simulink model "CACC_Model_5V"  (R2019b)
settings: Solver=ode45  StartTime=0.0  StopTime=20  FixedStep=0.01  MaxStep=0.001  RelTol=1e-3  EnableMultiTasking=on
InitFcn:
  | %% CACC Simulation Parameters
  | %% by M.Tolga EMIRLER ITU MEKAR
undefined symbols (not defined in the file): sigbuilder_block
libraries: simulink_need_slupdate x5, simulink x1
settings Model: Creator=Tolga  LastModifiedBy=subhajyotisarkar
settings DataIOCC: LimitDataPoints=on  SaveFormat=Array  SignalLoggingSaveFormat=ModelDataLogs  ReturnWorkspaceOutputs=off
settings OptimizationCC: ExpressionDepthLimit=2147483647  LifeSpan=inf
settings DebuggingCC: UnderspecifiedInitializationDetection=Classic  MergeDetectMultiDrivingBlocksExec=none  SolverPrmCheckMsg=warning  FcnCallInpInsideContextMsg=warning  StateNameClashWarn=warning  SFUnexpectedBacktrackingDiag=warning  SFNoUnconditionalDefaultTransitionDiag=warning  SFExecutionAtInitializationDiag=none  ArithmeticOperatorsInVariantConditions=warning
settings HardwareCC: ProdBitPerPointer=32  ProdBitPerSizeT=32  ProdBitPerPtrDiffT=32  ProdLargestAtomicFloat=None  ProdIntDivRoundTo=Undefined  ProdEndianess=Unspecified  ProdWordSize=32  ProdHWDeviceType=32-bit Generic
settings ModelReferenceCC: PropagateSignalLabelsOutOfModel=off
settings SFSimCC: SimUseLocalCustomCode=off  CustomCodeUndefinedFunction=UseInterfaceOnly
settings RTWCC: RTWUseLocalCustomCode=off
settings CodeAppCC: StateflowObjectComments=on
settings GRTTargetCC: TargetLangStandard=C89/C90 (ANSI)  GeneratePreprocessorConditionals=Disable all  CombineOutputUpdateFcns=off  GRTInterface=on
settings ConfigComp: CovMetricSettings=dw  CovHtmlReporting=on  CovSaveCumulativeToWorkspaceVar=on  CovSaveSingleToWorkspaceVar=on  CovExternalEMLEnable=off  CovSFcnEnable=off

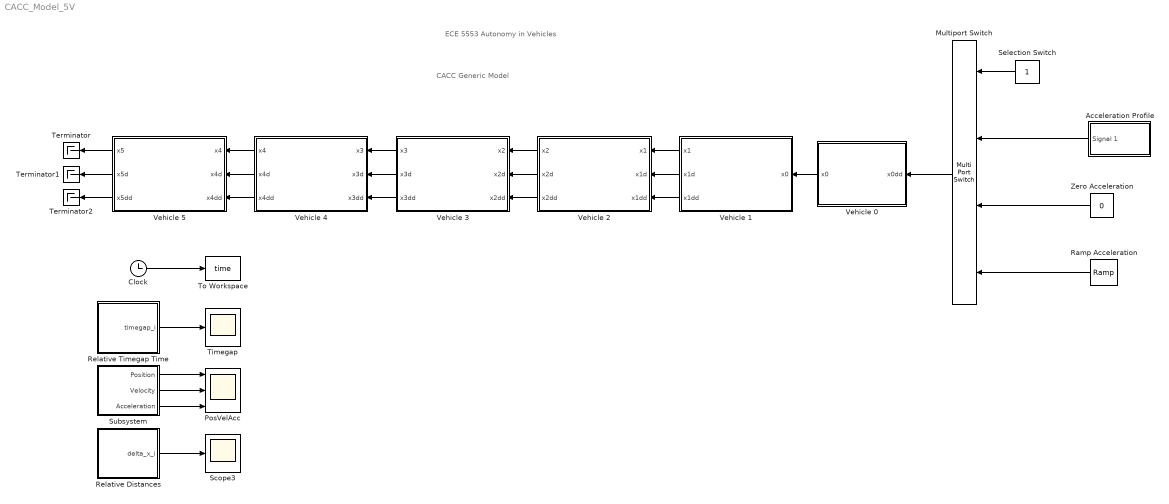
== system CACC_Model_5V ==
  note: ECE 5553 Autonomy in Vehicles
  note: CACC Generic Model
  Acceleration Profile : Subsystem  Tag=STV Subsys  LoadFcn=sigbuilder_block('load');  StartFcn=sigbuilder_block('start');  StopFcn=sigbuilder_block('stop');  ClipboardFcn=sigbuilder_block('clipboard');  mask(Sigbuilder block){tuvar=[0:10]}
      mask help: Sigbuilder GUI
      mask init:
      | if ~strcmp(get_param(bdroot(gcbh),'SimulationStatus'),'stopped') tuvar = sigbuilder_block('maskInit'); end
      settings: CopyFcn=sigbuilder_block('copy');  DeleteFcn=sigbuilder_block('delete');  ModelCloseFcn=sigbuilder_block('modelClose');  PreSaveFcn=sigbuilder_block('preSave');  PauseFcn=sigbuilder_block('pause')  ContinueFcn=sigbuilder_block('continue')  NameChangeFcn=sigbuilder_block('namechange');  OpenFcn=sigbuilder_block('open',[386.25 100.5 510.75 487.5 ]);  CloseFcn=sigbuilder_block('close');
      mask Display: plot(0, 0, 100, 100,[2, 2, 32, 32, 2], [68, 8, 8, 68, 68],[32, 2], [38, 38], [32, 19, 2],[53, 60, 44], [32, 17, 17, 2],[16, 16, 31, 31]);txt = getActiveGroup(gcbh);text(2, 100, txt,'verticalAlignment', 'top');
  Clock : Clock
  Multiport Switch : MultiPortSwitch
  PosVelAcc : Scope  NumInputPorts=3
  Ramp Acceleration : simulink/Sources/Ramp  slope=1  start=0  InitialOutput=40
  Relative Distances : Subsystem
  Relative Timegap Time : Subsystem
  Scope3 : Scope
  Selection Switch : Constant
  Subsystem : Subsystem
  Terminator : Terminator
  Terminator1 : Terminator
  Terminator2 : Terminator
  Timegap : Scope
  To Workspace : ToWorkspace  VariableName=time  SampleTime=-1
  Vehicle 0 : Subsystem  mask(INPUT BLOCK){x0in=250, V0in=25}
      mask prompts: x0in "Initial position (x0in)"; V0in "Initial velocity (V0in)"
      mask help: This block defines the input. Input (or disturbance) is the acceleration.
      mask Display:
      | disp('Input')
      | port_label('input',1,'a0')
      | port_label('output',1,'x0')
  Vehicle 1 : Subsystem  mask(VEHICLE #1 (GCDC Vehicle)){kG1=1.0, T1=0.5, phi1=0.1, theta1=0.3, hd1=0.6, L1=5, r1=30, x1in=200, V1in=25, CACC1=1, wK1=2.4}
      mask prompts: kG1 "Vehicle Model Gain (kG1)"; T1 "Vehicle Time Constant (T1)"; phi1 "Actuator (Internal) Delay (phi1) [s]"; theta1 "Communication System Delay (theta1) [s]"; hd1 "Headway time (hd1) [s]"; L1 "Vehicle length (L1) [m]"; r1 "Distance at standstill (r1) [m]"; x1in "Initial vehicle position (x1in) [m]"; V1in "Initial vehicle velocity (V1in) [m/sec]"; CACC1 "CACC On/Off [0 or 1]"; wK1 "Controller Gain (wK1)"
      mask help: Parameters for vehicle 1
      mask Display:
      | disp('Vehicle 1')
      | port_label('input',1,'x0')
      | port_label('output',1,'x1')
      | port_label('output',2,'V1')
      | port_label('output',3,'a1')
  Vehicle 2 : Subsystem  mask(VEHICLE #2){kG2=1.0, T2=0.5, phi2=0.1, theta2=0.3, hd2=0.6, L2=5, r2=30, x2in=150, V2in=25, CACC2=0, wK2=2.4}
      mask prompts: kG2 "Vehicle Model Gain (kG2)"; T2 "Vehicle Time Constant (T2)"; phi2 "Actuator (Internal) Delay (phi2) [s]"; theta2 "Communication System Delay (theta2) [s]"; hd2 "Headway time (hd2) [s]"; L2 "Vehicle length (L2) [m]"; r2 "Distance at standstill (r2) [m]"; x2in "Initial vehicle position (x2in) [m]"; V2in "Initial vehicle velocity (V2in) [m/sec]"; CACC2 "CACC On/Off [0 or 1]"; wK2 "Controller Gain (wK2)"
      mask help: Parameters for vehicle 2
      mask Display:
      | disp('Vehicle 2')
      | port_label('input',1,'x1')
      | port_label('input',2,'V1')
      | port_label('input',3,'a1')
      | port_label('output',1,'x2')
      | port_label('output',2,'V2')
      | port_label('output',3,'a2')
  Vehicle 3 : Subsystem  mask(VEHICLE #3){kG3=1.0, T3=0.5, phi3=0.1, theta3=0.3, hd3=0.6, L3=5, r3=30, x3in=100, V3in=25, CACC3=0, wK3=2.4}
      mask prompts: kG3 "Vehicle Model Gain (kG3)"; T3 "Vehicle Time Constant (T3)"; phi3 "Actuator (Internal) Delay (phi3) [s]"; theta3 "Communication System Delay (theta3) [s]"; hd3 "Headway time (hd3) [s]"; L3 "Vehicle length (L3) [m]"; r3 "Distance at standstill (r3) [m]"; x3in "Initial vehicle position (x3in) [m]"; V3in "Initial vehicle velocity (V3in) [m/sec]"; CACC3 "CACC On/Off [0 or 1]"; wK3 "Controller Gain (wK3)"
      mask help: Parameters for vehicle 3
      mask Display:
      | disp('Vehicle 3')
      | port_label('input',1,'x2')
      | port_label('input',2,'V2')
      | port_label('input',3,'a2')
      | port_label('output',1,'x3')
      | port_label('output',2,'V3')
      | port_label('output',3,'a3')
  Vehicle 4 : Subsystem  mask(VEHICLE #4){kG4=1.0, T4=0.5, phi4=0.1, theta4=0.3, hd4=0.6, L4=5, r4=30, x4in=50, V4in=25, CACC4=0, wK4=2.4}
      mask prompts: kG4 "Vehicle Model Gain (kG4)"; T4 "Vehicle Time Constant (T4)"; phi4 "Actuator (Internal) Delay (phi4) [s]"; theta4 "Communication System Delay (theta4) [s]"; hd4 "Headway time (hd4) [s]"; L4 "Vehicle length (L4) [m]"; r4 "Distance at standstill (r4) [m]"; x4in "Initial vehicle position (x4in) [m]"; V4in "Initial vehicle velocity (V4in) [m/sec]"; CACC4 "CACC On/Off [0 or 1]"; wK4 "Controller Gain (wK4)"
      mask help: Parameters for vehicle 4
      mask Display:
      | disp('Vehicle 4')
      | port_label('input',1,'x3')
      | port_label('input',2,'V3')
      | port_label('input',3,'a3')
      | port_label('output',1,'x4')
      | port_label('output',2,'V4')
      | port_label('output',3,'a4')
  Vehicle 5 : Subsystem  mask(VEHICLE #5){kG5=1.0, T5=0.5, phi5=0.1, theta5=0.3, hd5=0.6, L5=5, r5=30, x5in=0, V5in=25, CACC5=0, wK5=2.4}
      mask prompts: kG5 "Vehicle Model Gain (kG5)"; T5 "Vehicle Time Constant (T5)"; phi5 "Actuator (Internal) Delay (phi5) [s]"; theta5 "Communication System Delay (theta5) [s]"; hd5 "Headway time (hd5) [s]"; L5 "Vehicle length (L5) [m]"; r5 "Distance at standstill (r5) [m]"; x5in "Initial vehicle position (x5in) [m]"; V5in "Initial vehicle velocity (V5in) [m/sec]"; CACC5 "CACC On/Off [0 or 1]"; wK5 "Controller Gain (wK5)"
      mask help: Parameters for vehicle 5
      mask Display:
      | disp('Vehicle 5')
      | port_label('input',1,'x4')
      | port_label('input',2,'V4')
      | port_label('input',3,'a4')
      | port_label('output',1,'x5')
      | port_label('output',2,'V5')
      | port_label('output',3,'a5')
  Zero Acceleration : Constant  Value=0
  wires:
  Clock/1 -> To Workspace/1
  Relative Distances/1(delta_x_i) -> Scope3/1
  Vehicle 2/1(x2) -> Vehicle 3/1(x2)
  Vehicle 2/2(x2d) -> Vehicle 3/2(x2d)
  Vehicle 4/1(x4) -> Vehicle 5/1(x4)
  Vehicle 4/2(x4d) -> Vehicle 5/2(x4d)
  Vehicle 4/3(x4dd) -> Vehicle 5/3(x4dd)
  Vehicle 3/1(x3) -> Vehicle 4/1(x3)
  Vehicle 3/2(x3d) -> Vehicle 4/2(x3d)
  Vehicle 1/1(x1) -> Vehicle 2/1(x1)
  Vehicle 1/2(x1d) -> Vehicle 2/2(x1d)
  Vehicle 0/1(x0) -> Vehicle 1/1(x0)
  Ramp Acceleration/1 -> Multiport Switch/4
  Vehicle 1/3(x1dd) -> Vehicle 2/3(x1dd)
  Vehicle 2/3(x2dd) -> Vehicle 3/3(x2dd)
  Vehicle 3/3(x3dd) -> Vehicle 4/3(x3dd)
  Acceleration Profile/1(Signal 1) -> Multiport Switch/2
  Zero Acceleration/1 -> Multiport Switch/3
  Vehicle 5/1(x5) -> Terminator/1
  Vehicle 5/2(x5d) -> Terminator1/1
  Vehicle 5/3(x5dd) -> Terminator2/1
  Relative Timegap Time/1(timegap_i) -> Timegap/1
  Selection Switch/1 -> Multiport Switch/1
  Multiport Switch/1 -> Vehicle 0/1(x0dd)
  Subsystem/1(Position) -> PosVelAcc/1
  Subsystem/2(Velocity) -> PosVelAcc/2
  Subsystem/3(Acceleration) -> PosVelAcc/3

== system CACC_Model_5V/Acceleration Profile ==
  Demux : Demux  Tag=STV Demux  Outputs=1
  FromWs : FromWorkspace  Tag=STV FromWs  VariableName=tuvar  SampleTime=0
      SigBuilderData=|
      | common.afterFinalStr = 'Extrapolate'
      | common.sampleTime = 0
      | dataSet.timeRange = [0 50]
      | dataSet.name = 'Group 1'
      | sbobj.Groups.Name = 'Group 1'
      | sbobj.Groups.Signals.Name = 'Signal 1'
      | sbobj.Groups.Signals.XData = [0 5 10 15 25 30 35 40 50]
      | sbobj.Groups.Signals.YData = [0 1 1 0 0 -1 -1 0 0]
      | sbobj.Groups.TimeRange = [0 50]
  Signal 1 : Outport  Tag=STV Outport  VectorParamsAs1DForOutWhenUnconnected=off
  wires:
  Demux/1 -> Signal 1/1
  FromWs/1 -> Demux/1

== system CACC_Model_5V/Relative Distances ==
  Mux2 : Mux
  Sum{,1..3} (4 alike) : Sum  Inputs=|+-
  delta_x_i : Outport  VectorParamsAs1DForOutWhenUnconnected=off
  wires:
  [x1] -> Sum/1
  [x2] -> Sum/2, Sum1/1
  [x3] -> Sum1/2, Sum2/1
  Sum/1 -> Mux2/1
  Sum1/1 -> Mux2/2
  Sum2/1 -> Mux2/3
  Mux2/1 -> delta_x_i/1
  Sum3/1 -> Mux2/4
  [x5] -> Sum3/2
  [x4] -> Sum3/1, Sum2/2

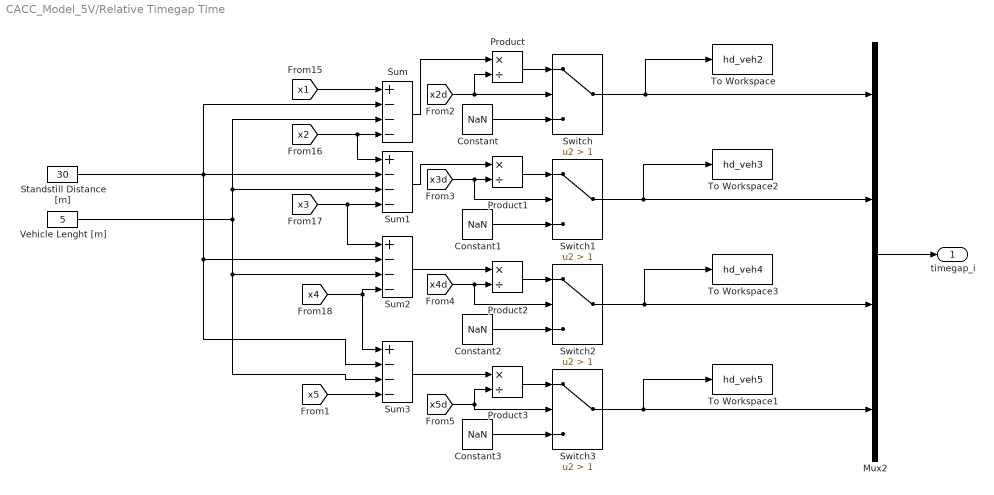
== system CACC_Model_5V/Relative Timegap Time ==
  Constant{,1..3} (4 alike) : Constant  Value=NaN
  Mux2 : Mux
  Product{,1..3} (4 alike) : Product  Inputs=*/
  Standstill Distance [m] : Constant  Value=30
  Sum{,1..3} (4 alike) : Sum  Inputs=+---
  Switch{,1..3} (4 alike) : Switch  Criteria=u2 > Threshold  Threshold=1
  To Workspace : ToWorkspace  VariableName=hd_veh2  SampleTime=-1
  To Workspace1 : ToWorkspace  VariableName=hd_veh5  SampleTime=-1
  To Workspace2 : ToWorkspace  VariableName=hd_veh3  SampleTime=-1
  To Workspace3 : ToWorkspace  VariableName=hd_veh4  SampleTime=-1
  Vehicle Lenght [m] : Constant  Value=5
  timegap_i : Outport  VectorParamsAs1DForOutWhenUnconnected=off
  wires:
  [x4] -> Sum3/1, Sum2/4
  [x5] -> Sum3/4
  Mux2/1 -> timegap_i/1
  Sum/1 -> Product/1
  [x3] -> Sum2/1, Sum1/4
  [x2] -> Sum1/1, Sum/4
  [x1] -> Sum/1
  Product/1 -> Switch/1
  [x2d] -> Switch/2, Product/2
  Constant/1 -> Switch/3
  Switch/1 -> Mux2/1, To Workspace/1
  Constant1/1 -> Switch1/3
  [x3d] -> Switch1/2, Product1/2
  Product1/1 -> Switch1/1
  Sum1/1 -> Product1/1
  Sum2/1 -> Product2/1
  Product2/1 -> Switch2/1
  [x4d] -> Switch2/2, Product2/2
  Constant2/1 -> Switch2/3
  Constant3/1 -> Switch3/3
  [x5d] -> Switch3/2, Product3/2
  Product3/1 -> Switch3/1
  Sum3/1 -> Product3/1
  Switch1/1 -> To Workspace2/1, Mux2/2
  Switch3/1 -> To Workspace1/1, Mux2/4
  Switch2/1 -> To Workspace3/1, Mux2/3
  Standstill Distance [m]/1 -> Sum3/2, Sum2/2, Sum1/2, Sum/2
  Vehicle Lenght [m]/1 -> Sum3/3, Sum2/3, Sum1/3, Sum/3

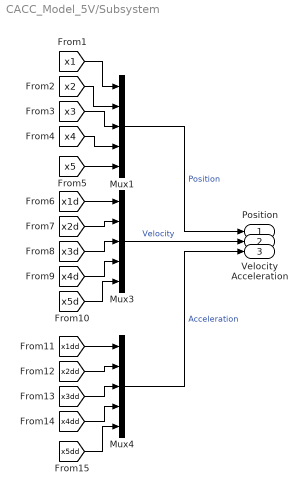
== system CACC_Model_5V/Subsystem ==
  Mux1 : Mux  Inputs=5
  Mux3 : Mux  Inputs=5
  Mux4 : Mux  Inputs=5
  Position : Outport  VectorParamsAs1DForOutWhenUnconnected=off
  Velocity : Outport  Port=2  VectorParamsAs1DForOutWhenUnconnected=off
  Acceleration : Outport  Port=3  VectorParamsAs1DForOutWhenUnconnected=off
  wires:
  Mux1/1 -> Position/1  "Position"
  Mux3/1 -> Velocity/1  "Velocity"
  Mux4/1 -> Acceleration/1  "Acceleration"
  [x2dd] -> Mux4/2
  [x2] -> Mux1/2
  [x1dd] -> Mux4/1
  [x4d] -> Mux3/4
  [x1] -> Mux1/1
  [x4] -> Mux1/4
  [x1d] -> Mux3/1
  [x3d] -> Mux3/3
  [x4dd] -> Mux4/4
  [x3] -> Mux1/3
  [x2d] -> Mux3/2
  [x3dd] -> Mux4/3
  [x5dd] -> Mux4/5
  [x5d] -> Mux3/5
  [x5] -> Mux1/5

== system CACC_Model_5V/Vehicle 0 ==
  x0dd : Inport
  Integrator : Integrator  InitialCondition=V0in
  Integrator1 : Integrator  InitialCondition=x0in
  To Workspace : ToWorkspace  VariableName=x0dd  SampleTime=-1
  To Workspace1 : ToWorkspace  VariableName=x0d  SampleTime=-1
  To Workspace2 : ToWorkspace  VariableName=x0  SampleTime=-1
  x0 : Outport  VectorParamsAs1DForOutWhenUnconnected=off
  wires:
  Integrator/1 -> Integrator1/1, To Workspace1/1
  x0dd/1 -> Integrator/1, To Workspace/1
  Integrator1/1 -> x0/1, To Workspace2/1

== system CACC_Model_5V/Vehicle 1 ==
  note: a
  note: e1
  note: Spacing Error
  x0 : Inport
  ACC Signal Measurement Delay : TransportDelay  DelayTime=0
  PD Controller : simulink_need_slupdate/PID Controller  P=wK1^2  I=0  D=wK1
      settings: SourceProductName=Simulink
  Spacing Policy : Subsystem
  Vehicle 1 : Subsystem
  x1 : Outport  VectorParamsAs1DForOutWhenUnconnected=off
  x1d : Outport  Port=2  VectorParamsAs1DForOutWhenUnconnected=off
  x1dd : Outport  Port=3  VectorParamsAs1DForOutWhenUnconnected=off
  wires:
  Vehicle 1/3(x1dd) -> x1dd/1
  Vehicle 1/2(x1d) -> x1d/1, Spacing Policy/3(x2d)
  Vehicle 1/1(x1) -> x1/1, Spacing Policy/2(x1)
  Spacing Policy/1(e1) -> PD Controller/1
  x0/1 -> ACC Signal Measurement Delay/1
  PD Controller/1 -> Vehicle 1/1(a_cont1)
  ACC Signal Measurement Delay/1 -> Spacing Policy/1(x0)

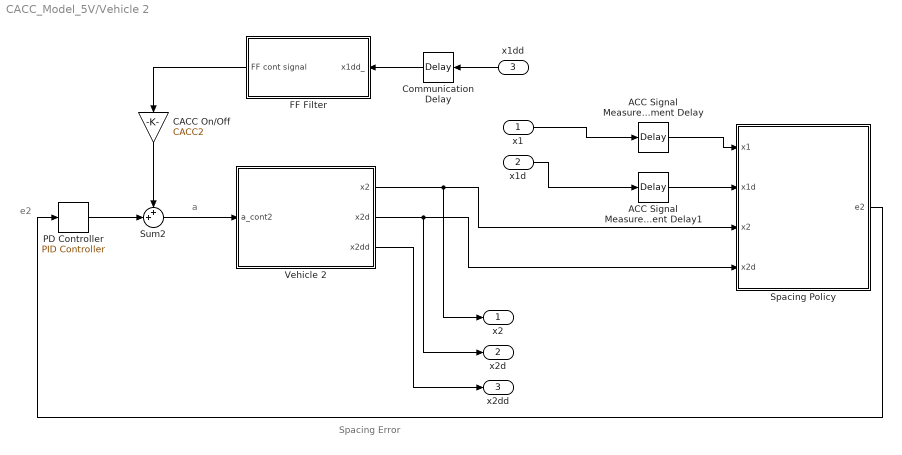
== system CACC_Model_5V/Vehicle 2 ==
  note: Spacing Error
  note: e2
  note: a
  x1 : Inport
  x1d : Inport  Port=2
  x1dd : Inport  Port=3
  ACC Signal Measurement Delay : TransportDelay  DelayTime=0
  ACC Signal Measurement Delay1 : TransportDelay  DelayTime=0
  CACC On/Off : Gain  Gain=CACC2
  Communication Delay : TransportDelay  DelayTime=theta2
  FF Filter : Subsystem
  PD Controller : simulink_need_slupdate/PID Controller  P=wK2*wK2  I=0  D=wK2
      settings: SourceProductName=Simulink
  Spacing Policy : Subsystem
  Sum2 : Sum  Inputs=++|
  Vehicle 2 : Subsystem
  x2 : Outport  VectorParamsAs1DForOutWhenUnconnected=off
  x2d : Outport  Port=2  VectorParamsAs1DForOutWhenUnconnected=off
  x2dd : Outport  Port=3  VectorParamsAs1DForOutWhenUnconnected=off
  wires:
  PD Controller/1 -> Sum2/2
  Sum2/1 -> Vehicle 2/1(a_cont2)
  x1dd/1 -> Communication Delay/1
  Communication Delay/1 -> FF Filter/1(x1dd_)
  x1/1 -> ACC Signal Measurement Delay/1
  Spacing Policy/1(e2) -> PD Controller/1
  x1d/1 -> ACC Signal Measurement Delay1/1
  Vehicle 2/1(x2) -> Spacing Policy/3(x2), x2/1
  Vehicle 2/2(x2d) -> Spacing Policy/4(x2d), x2d/1
  Vehicle 2/3(x2dd) -> x2dd/1
  FF Filter/1(FF cont signal) -> CACC On/Off/1
  CACC On/Off/1 -> Sum2/1
  ACC Signal Measurement Delay/1 -> Spacing Policy/1(x1)
  ACC Signal Measurement Delay1/1 -> Spacing Policy/2(x1d)

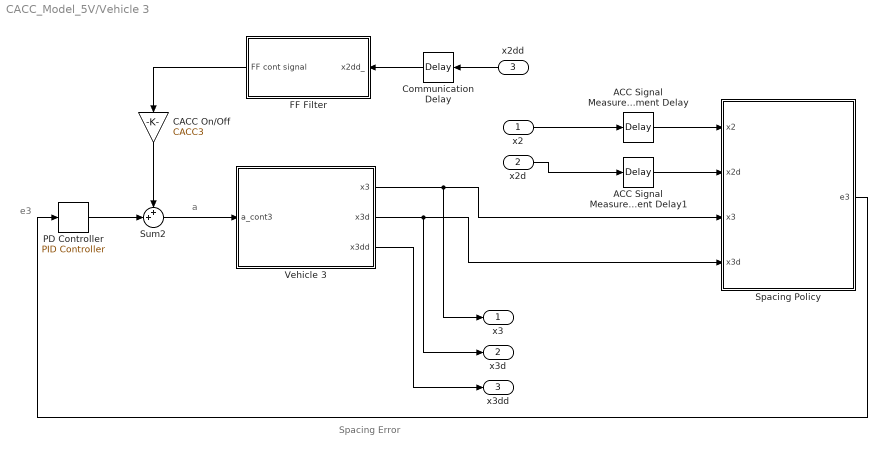
== system CACC_Model_5V/Vehicle 3 ==
  note: a
  note: e3
  note: Spacing Error
  x2 : Inport
  x2d : Inport  Port=2
  x2dd : Inport  Port=3
  ACC Signal Measurement Delay : TransportDelay  DelayTime=0
  ACC Signal Measurement Delay1 : TransportDelay  DelayTime=0
  CACC On/Off : Gain  Gain=CACC3
  Communication Delay : TransportDelay  DelayTime=theta3
  FF Filter : Subsystem
  PD Controller : simulink_need_slupdate/PID Controller  P=wK3*wK3  I=0  D=wK3
      settings: SourceProductName=Simulink
  Spacing Policy : Subsystem
  Sum2 : Sum  Inputs=++|
  Vehicle 3 : Subsystem
  x3 : Outport  VectorParamsAs1DForOutWhenUnconnected=off
  x3d : Outport  Port=2  VectorParamsAs1DForOutWhenUnconnected=off
  x3dd : Outport  Port=3  VectorParamsAs1DForOutWhenUnconnected=off
  wires:
  CACC On/Off/1 -> Sum2/1
  FF Filter/1(FF cont signal) -> CACC On/Off/1
  Vehicle 3/3(x3dd) -> x3dd/1
  Vehicle 3/2(x3d) -> x3d/1, Spacing Policy/4(x3d)
  Vehicle 3/1(x3) -> x3/1, Spacing Policy/3(x3)
  x2d/1 -> ACC Signal Measurement Delay1/1
  Spacing Policy/1(e3) -> PD Controller/1
  x2/1 -> ACC Signal Measurement Delay/1
  Communication Delay/1 -> FF Filter/1(x2dd_)
  x2dd/1 -> Communication Delay/1
  Sum2/1 -> Vehicle 3/1(a_cont3)
  PD Controller/1 -> Sum2/2
  ACC Signal Measurement Delay/1 -> Spacing Policy/1(x2)
  ACC Signal Measurement Delay1/1 -> Spacing Policy/2(x2d)

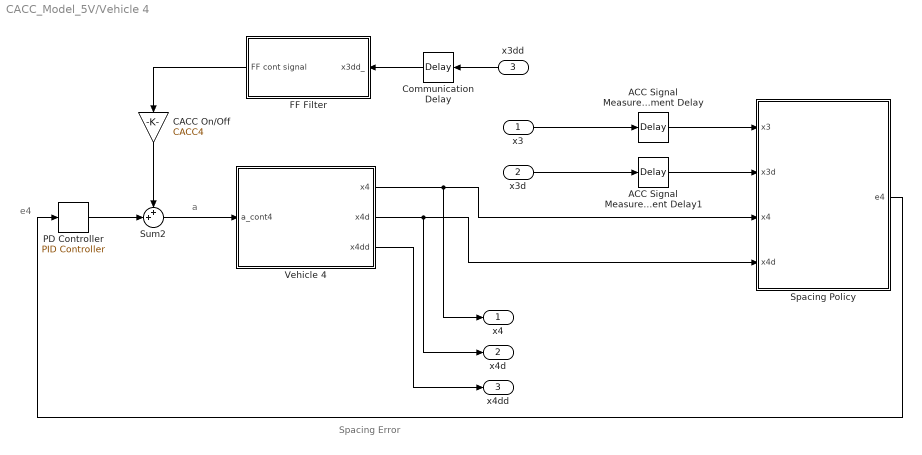
== system CACC_Model_5V/Vehicle 4 ==
  note: a
  note: e4
  note: Spacing Error
  x3 : Inport
  x3d : Inport  Port=2
  x3dd : Inport  Port=3
  ACC Signal Measurement Delay : TransportDelay  DelayTime=0
  ACC Signal Measurement Delay1 : TransportDelay  DelayTime=0
  CACC On/Off : Gain  Gain=CACC4
  Communication Delay : TransportDelay  DelayTime=theta4
  FF Filter : Subsystem
  PD Controller : simulink_need_slupdate/PID Controller  P=wK4*wK4  I=0  D=wK4
      settings: SourceProductName=Simulink
  Spacing Policy : Subsystem
  Sum2 : Sum  Inputs=++|
  Vehicle 4 : Subsystem
  x4 : Outport  VectorParamsAs1DForOutWhenUnconnected=off
  x4d : Outport  Port=2  VectorParamsAs1DForOutWhenUnconnected=off
  x4dd : Outport  Port=3  VectorParamsAs1DForOutWhenUnconnected=off
  wires:
  CACC On/Off/1 -> Sum2/1
  FF Filter/1(FF cont signal) -> CACC On/Off/1
  Vehicle 4/3(x4dd) -> x4dd/1
  Vehicle 4/2(x4d) -> x4d/1, Spacing Policy/4(x4d)
  Vehicle 4/1(x4) -> x4/1, Spacing Policy/3(x4)
  x3d/1 -> ACC Signal Measurement Delay1/1
  Spacing Policy/1(e4) -> PD Controller/1
  x3/1 -> ACC Signal Measurement Delay/1
  Communication Delay/1 -> FF Filter/1(x3dd_)
  x3dd/1 -> Communication Delay/1
  Sum2/1 -> Vehicle 4/1(a_cont4)
  PD Controller/1 -> Sum2/2
  ACC Signal Measurement Delay1/1 -> Spacing Policy/2(x3d)
  ACC Signal Measurement Delay/1 -> Spacing Policy/1(x3)

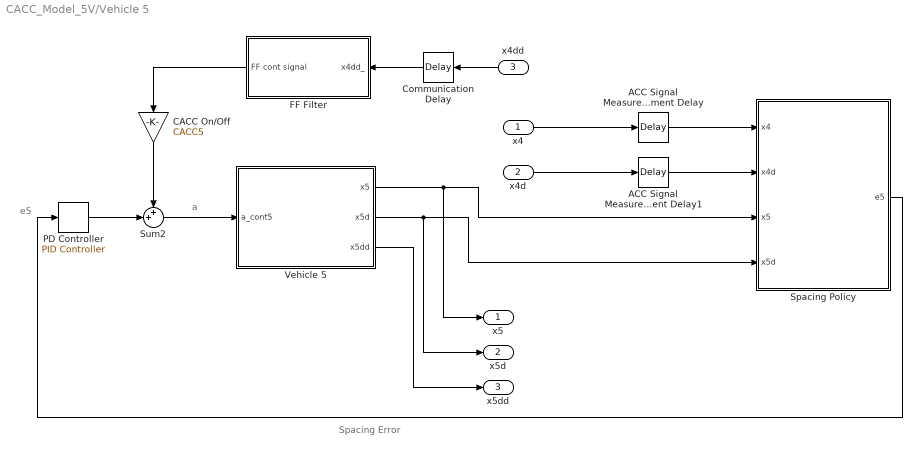
== system CACC_Model_5V/Vehicle 5 ==
  note: Spacing Error
  note: e5
  note: a
  x4 : Inport
  x4d : Inport  Port=2
  x4dd : Inport  Port=3
  ACC Signal Measurement Delay : TransportDelay  DelayTime=0
  ACC Signal Measurement Delay1 : TransportDelay  DelayTime=0
  CACC On/Off : Gain  Gain=CACC5
  Communication Delay : TransportDelay  DelayTime=theta5
  FF Filter : Subsystem
  PD Controller : simulink_need_slupdate/PID Controller  P=wK5*wK5  I=0  D=wK5
      settings: SourceProductName=Simulink
  Spacing Policy : Subsystem
  Sum2 : Sum  Inputs=++|
  Vehicle 5 : Subsystem
  x5 : Outport  VectorParamsAs1DForOutWhenUnconnected=off
  x5d : Outport  Port=2  VectorParamsAs1DForOutWhenUnconnected=off
  x5dd : Outport  Port=3  VectorParamsAs1DForOutWhenUnconnected=off
  wires:
  ACC Signal Measurement Delay/1 -> Spacing Policy/1(x4)
  ACC Signal Measurement Delay1/1 -> Spacing Policy/2(x4d)
  PD Controller/1 -> Sum2/2
  Sum2/1 -> Vehicle 5/1(a_cont5)
  x4dd/1 -> Communication Delay/1
  Communication Delay/1 -> FF Filter/1(x4dd_)
  x4/1 -> ACC Signal Measurement Delay/1
  Spacing Policy/1(e5) -> PD Controller/1
  x4d/1 -> ACC Signal Measurement Delay1/1
  Vehicle 5/1(x5) -> Spacing Policy/3(x5), x5/1
  Vehicle 5/2(x5d) -> Spacing Policy/4(x5d), x5d/1
  Vehicle 5/3(x5dd) -> x5dd/1
  FF Filter/1(FF cont signal) -> CACC On/Off/1
  CACC On/Off/1 -> Sum2/1

== system CACC_Model_5V/Vehicle 1/Spacing Policy ==
  x0 : Inport
  x1 : Inport  Port=2
  x2d : Inport  Port=3
  Constant : Constant  Value=r1
  Constant1 : Constant  Value=L1
  Headway Time : Gain  Gain=hd1
  Sum : Sum  Inputs=+----
  e1 : Outport  VectorParamsAs1DForOutWhenUnconnected=off
  wires:
  x2d/1 -> Headway Time/1
  Headway Time/1 -> Sum/3
  Sum/1 -> e1/1
  x1/1 -> Sum/2
  x0/1 -> Sum/1
  Constant1/1 -> Sum/5
  Constant/1 -> Sum/4

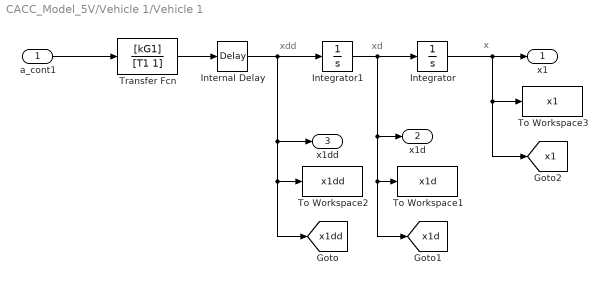
== system CACC_Model_5V/Vehicle 1/Vehicle 1 ==
  note: xdd
  note: xd
  note: x
  a_cont1 : Inport
  Integrator : Integrator  InitialCondition=x1in
  Integrator1 : Integrator  InitialCondition=V1in
  Internal Delay : TransportDelay  DelayTime=phi1
  To Workspace1 : ToWorkspace  VariableName=x1d  SampleTime=-1
  To Workspace2 : ToWorkspace  VariableName=x1dd  SampleTime=-1
  To Workspace3 : ToWorkspace  VariableName=x1  SampleTime=-1
  Transfer Fcn : TransferFcn  Numerator=[kG1]  Denominator=[T1 1]
  x1 : Outport  VectorParamsAs1DForOutWhenUnconnected=off
  x1d : Outport  Port=2  VectorParamsAs1DForOutWhenUnconnected=off
  x1dd : Outport  Port=3  VectorParamsAs1DForOutWhenUnconnected=off
  tag scope: x1=global, x1d=global, x1dd=global
  wires:
  Integrator/1 -> [x1], To Workspace3/1, x1/1
  a_cont1/1 -> Transfer Fcn/1
  Transfer Fcn/1 -> Internal Delay/1
  Internal Delay/1 -> [x1dd], To Workspace2/1, x1dd/1, Integrator1/1
  Integrator1/1 -> [x1d], To Workspace1/1, x1d/1, Integrator/1

== system CACC_Model_5V/Vehicle 2/FF Filter ==
  x1dd_ : Inport
  Feedforward Filter : TransferFcn  Numerator=[T2 1]  Denominator=kG2*[hd2 1]
  FF cont signal : Outport  VectorParamsAs1DForOutWhenUnconnected=off
  wires:
  x1dd_/1 -> Feedforward Filter/1
  Feedforward Filter/1 -> FF cont signal/1

== system CACC_Model_5V/Vehicle 2/Spacing Policy ==
  x1 : Inport
  x1d : Inport  Port=2
  x2 : Inport  Port=3
  x2d : Inport  Port=4
  Constant : Constant  Value=r2
  Constant1 : Constant  Value=L2
  Headway Time : Gain  Gain=hd2
  Sum : Sum  Inputs=+----
  Terminator : Terminator
  e2 : Outport  VectorParamsAs1DForOutWhenUnconnected=off
  wires:
  Constant/1 -> Sum/4
  Constant1/1 -> Sum/5
  x1/1 -> Sum/1
  x2/1 -> Sum/2
  Sum/1 -> e2/1
  x1d/1 -> Terminator/1
  Headway Time/1 -> Sum/3
  x2d/1 -> Headway Time/1

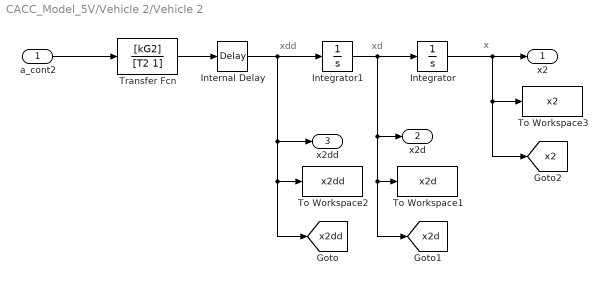
== system CACC_Model_5V/Vehicle 2/Vehicle 2 ==
  note: x
  note: xd
  note: xdd
  a_cont2 : Inport
  Integrator : Integrator  InitialCondition=x2in
  Integrator1 : Integrator  InitialCondition=V2in
  Internal Delay : TransportDelay  DelayTime=phi2
  To Workspace1 : ToWorkspace  VariableName=x2d  SampleTime=-1
  To Workspace2 : ToWorkspace  VariableName=x2dd  SampleTime=-1
  To Workspace3 : ToWorkspace  VariableName=x2  SampleTime=-1
  Transfer Fcn : TransferFcn  Numerator=[kG2]  Denominator=[T2 1]
  x2 : Outport  VectorParamsAs1DForOutWhenUnconnected=off
  x2d : Outport  Port=2  VectorParamsAs1DForOutWhenUnconnected=off
  x2dd : Outport  Port=3  VectorParamsAs1DForOutWhenUnconnected=off
  tag scope: x2=global, x2d=global, x2dd=global
  wires:
  Integrator1/1 -> Integrator/1, x2d/1, To Workspace1/1, [x2d]
  Internal Delay/1 -> Integrator1/1, x2dd/1, To Workspace2/1, [x2dd]
  Transfer Fcn/1 -> Internal Delay/1
  a_cont2/1 -> Transfer Fcn/1
  Integrator/1 -> x2/1, To Workspace3/1, [x2]

== system CACC_Model_5V/Vehicle 3/FF Filter ==
  x2dd_ : Inport
  Feedforward Filter : TransferFcn  Numerator=[T3 1]  Denominator=kG3*[hd3 1]
  FF cont signal : Outport  VectorParamsAs1DForOutWhenUnconnected=off
  wires:
  Feedforward Filter/1 -> FF cont signal/1
  x2dd_/1 -> Feedforward Filter/1

== system CACC_Model_5V/Vehicle 3/Spacing Policy ==
  x2 : Inport
  x2d : Inport  Port=2
  x3 : Inport  Port=3
  x3d : Inport  Port=4
  Constant : Constant  Value=r3
  Constant1 : Constant  Value=L3
  Headway Time : Gain  Gain=hd3
  Sum : Sum  Inputs=+----
  Terminator : Terminator
  e3 : Outport  VectorParamsAs1DForOutWhenUnconnected=off
  wires:
  x3d/1 -> Headway Time/1
  Headway Time/1 -> Sum/3
  x2d/1 -> Terminator/1
  Sum/1 -> e3/1
  x3/1 -> Sum/2
  x2/1 -> Sum/1
  Constant1/1 -> Sum/5
  Constant/1 -> Sum/4

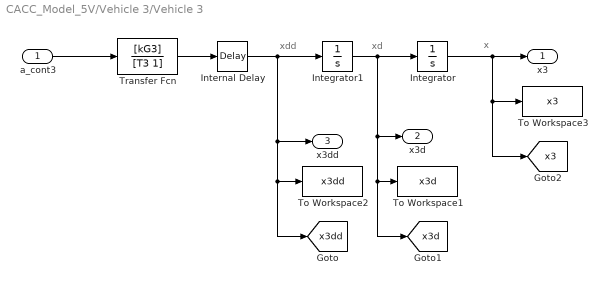
== system CACC_Model_5V/Vehicle 3/Vehicle 3 ==
  note: xdd
  note: xd
  note: x
  a_cont3 : Inport
  Integrator : Integrator  InitialCondition=x3in
  Integrator1 : Integrator  InitialCondition=V3in
  Internal Delay : TransportDelay  DelayTime=phi3
  To Workspace1 : ToWorkspace  VariableName=x3d  SampleTime=-1
  To Workspace2 : ToWorkspace  VariableName=x3dd  SampleTime=-1
  To Workspace3 : ToWorkspace  VariableName=x3  SampleTime=-1
  Transfer Fcn : TransferFcn  Numerator=[kG3]  Denominator=[T3 1]
  x3 : Outport  VectorParamsAs1DForOutWhenUnconnected=off
  x3d : Outport  Port=2  VectorParamsAs1DForOutWhenUnconnected=off
  x3dd : Outport  Port=3  VectorParamsAs1DForOutWhenUnconnected=off
  tag scope: x3=global, x3d=global, x3dd=global
  wires:
  Integrator/1 -> [x3], To Workspace3/1, x3/1
  a_cont3/1 -> Transfer Fcn/1
  Transfer Fcn/1 -> Internal Delay/1
  Internal Delay/1 -> [x3dd], To Workspace2/1, x3dd/1, Integrator1/1
  Integrator1/1 -> [x3d], To Workspace1/1, x3d/1, Integrator/1

== system CACC_Model_5V/Vehicle 4/FF Filter ==
  x3dd_ : Inport
  Feedforward Filter : TransferFcn  Numerator=[T4 1]  Denominator=kG4*[hd4 1]
  FF cont signal : Outport  VectorParamsAs1DForOutWhenUnconnected=off
  wires:
  Feedforward Filter/1 -> FF cont signal/1
  x3dd_/1 -> Feedforward Filter/1

== system CACC_Model_5V/Vehicle 4/Spacing Policy ==
  x3 : Inport
  x3d : Inport  Port=2
  x4 : Inport  Port=3
  x4d : Inport  Port=4
  Constant : Constant  Value=r4
  Constant1 : Constant  Value=L4
  Headway Time : Gain  Gain=hd4
  Sum : Sum  Inputs=+----
  Terminator : Terminator
  e4 : Outport  VectorParamsAs1DForOutWhenUnconnected=off
  wires:
  x4d/1 -> Headway Time/1
  Headway Time/1 -> Sum/3
  x3d/1 -> Terminator/1
  Sum/1 -> e4/1
  x4/1 -> Sum/2
  x3/1 -> Sum/1
  Constant1/1 -> Sum/5
  Constant/1 -> Sum/4

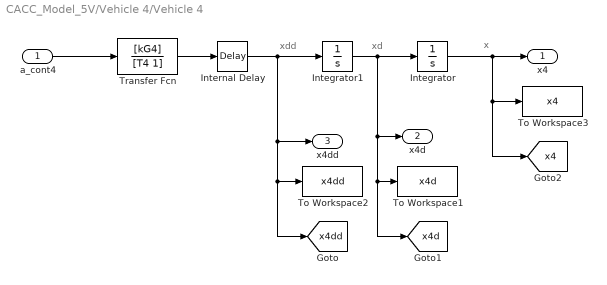
== system CACC_Model_5V/Vehicle 4/Vehicle 4 ==
  note: xdd
  note: xd
  note: x
  a_cont4 : Inport
  Integrator : Integrator  InitialCondition=x4in
  Integrator1 : Integrator  InitialCondition=V4in
  Internal Delay : TransportDelay  DelayTime=phi4
  To Workspace1 : ToWorkspace  VariableName=x4d  SampleTime=-1
  To Workspace2 : ToWorkspace  VariableName=x4dd  SampleTime=-1
  To Workspace3 : ToWorkspace  VariableName=x4  SampleTime=-1
  Transfer Fcn : TransferFcn  Numerator=[kG4]  Denominator=[T4 1]
  x4 : Outport  VectorParamsAs1DForOutWhenUnconnected=off
  x4d : Outport  Port=2  VectorParamsAs1DForOutWhenUnconnected=off
  x4dd : Outport  Port=3  VectorParamsAs1DForOutWhenUnconnected=off
  tag scope: x4=global, x4d=global, x4dd=global
  wires:
  Integrator/1 -> [x4], To Workspace3/1, x4/1
  a_cont4/1 -> Transfer Fcn/1
  Transfer Fcn/1 -> Internal Delay/1
  Internal Delay/1 -> [x4dd], To Workspace2/1, x4dd/1, Integrator1/1
  Integrator1/1 -> [x4d], To Workspace1/1, x4d/1, Integrator/1

== system CACC_Model_5V/Vehicle 5/FF Filter ==
  x4dd_ : Inport
  Feedforward Filter : TransferFcn  Numerator=[T5 1]  Denominator=kG5*[hd5 1]
  FF cont signal : Outport  VectorParamsAs1DForOutWhenUnconnected=off
  wires:
  x4dd_/1 -> Feedforward Filter/1
  Feedforward Filter/1 -> FF cont signal/1

== system CACC_Model_5V/Vehicle 5/Spacing Policy ==
  x4 : Inport
  x4d : Inport  Port=2
  x5 : Inport  Port=3
  x5d : Inport  Port=4
  Constant : Constant  Value=r5
  Constant1 : Constant  Value=L5
  Headway Time : Gain  Gain=hd5
  Sum : Sum  Inputs=+----
  Terminator : Terminator
  e5 : Outport  VectorParamsAs1DForOutWhenUnconnected=off
  wires:
  Constant/1 -> Sum/4
  Constant1/1 -> Sum/5
  x4/1 -> Sum/1
  x5/1 -> Sum/2
  Sum/1 -> e5/1
  x4d/1 -> Terminator/1
  Headway Time/1 -> Sum/3
  x5d/1 -> Headway Time/1

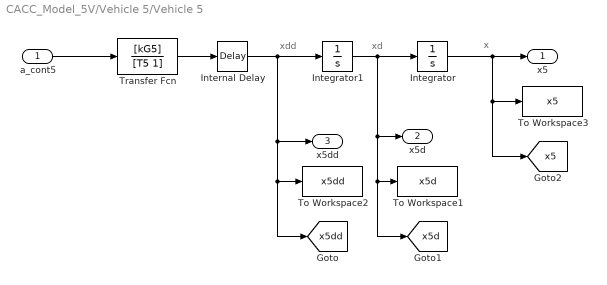
== system CACC_Model_5V/Vehicle 5/Vehicle 5 ==
  note: x
  note: xd
  note: xdd
  a_cont5 : Inport
  Integrator : Integrator  InitialCondition=x5in
  Integrator1 : Integrator  InitialCondition=V5in
  Internal Delay : TransportDelay  DelayTime=phi5
  To Workspace1 : ToWorkspace  VariableName=x5d  SampleTime=-1
  To Workspace2 : ToWorkspace  VariableName=x5dd  SampleTime=-1
  To Workspace3 : ToWorkspace  VariableName=x5  SampleTime=-1
  Transfer Fcn : TransferFcn  Numerator=[kG5]  Denominator=[T5 1]
  x5 : Outport  VectorParamsAs1DForOutWhenUnconnected=off
  x5d : Outport  Port=2  VectorParamsAs1DForOutWhenUnconnected=off
  x5dd : Outport  Port=3  VectorParamsAs1DForOutWhenUnconnected=off
  tag scope: x5=global, x5d=global, x5dd=global
  wires:
  Integrator1/1 -> Integrator/1, x5d/1, To Workspace1/1, [x5d]
  Internal Delay/1 -> Integrator1/1, x5dd/1, To Workspace2/1, [x5dd]
  Transfer Fcn/1 -> Internal Delay/1
  a_cont5/1 -> Transfer Fcn/1
  Integrator/1 -> x5/1, To Workspace3/1, [x5]
